simulink subsystem "subsistema_motores_bueno"  (R2023b)
settings: Solver=VariableStepAuto  StartTime=0.0  StopTime=10.0  RelTol=1e-3
libraries: arduinolib x6
settings Model: Creator=Usuario_UMA  LastModifiedBy=Usuario_UMA

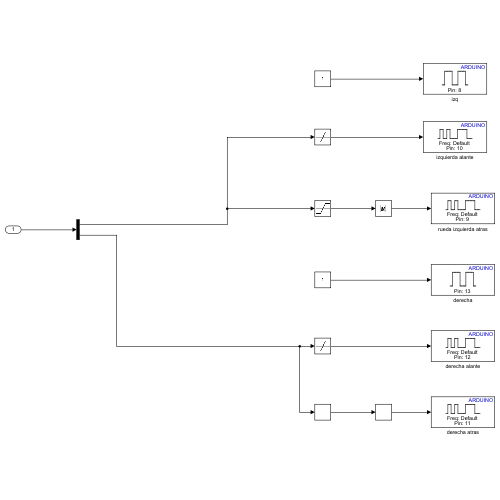
[thumbnail: Simulink's stored preview of the top-level diagram]
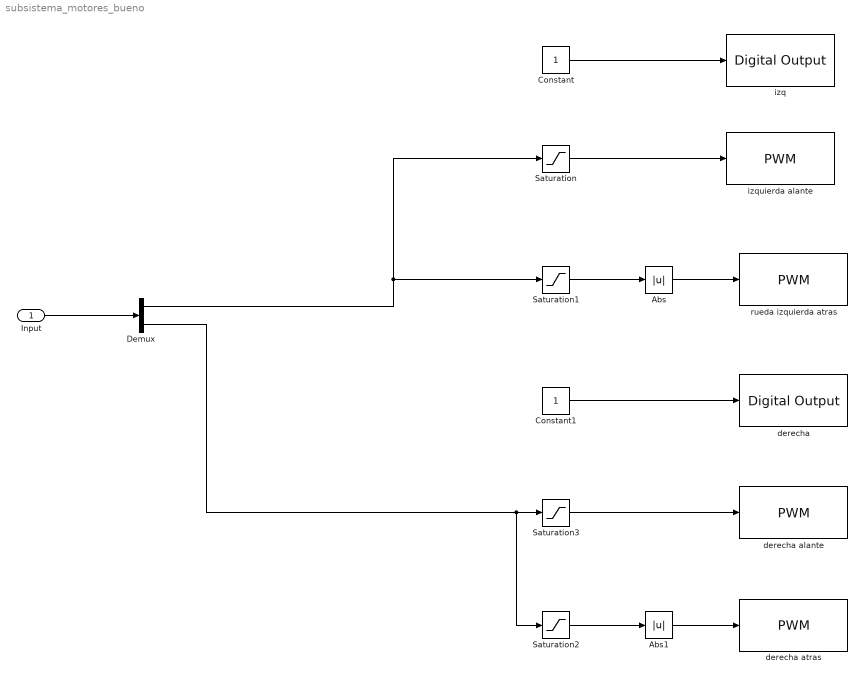
== system subsistema_motores_bueno ==
  Input : Inport
  Abs : Abs  SaturateOnIntegerOverflow=off
  Abs1 : Abs  SaturateOnIntegerOverflow=off
  Constant : Constant
  Constant1 : Constant
  Demux : Demux  Outputs=2
  Saturation : Saturate  UpperLimit=255  LowerLimit=0
  Saturation1 : Saturate  UpperLimit=0  LowerLimit=-255
  Saturation2 : Saturate  UpperLimit=0  LowerLimit=-255
  Saturation3 : Saturate  UpperLimit=255  LowerLimit=0
  derecha : arduinolib/Digital Output  pinNumber=13  Direction=output  blockPlatform=arduino
  derecha alante : arduinolib/PWM  pinNumber=12  frequencyType=Default  desiredFrequency=490.2  achievableFrequency=490.2
  derecha atras : arduinolib/PWM  pinNumber=11  frequencyType=Default  desiredFrequency=490.2  achievableFrequency=490.2
  izq : arduinolib/Digital Output  pinNumber=8  Direction=output  blockPlatform=arduino
  izquierda alante : arduinolib/PWM  pinNumber=10  frequencyType=Default  desiredFrequency=490.2  achievableFrequency=490.2
  rueda izquierda atras : arduinolib/PWM  pinNumber=9  frequencyType=Default  desiredFrequency=490.2  achievableFrequency=490.2
  wires:
  Saturation/1 -> izquierda alante/1
  Abs/1 -> rueda izquierda atras/1
  Demux/2 -> Saturation2/1, Saturation3/1
  Input/1 -> Demux/1
  Demux/1 -> Saturation/1, Saturation1/1
  Saturation1/1 -> Abs/1
  Saturation3/1 -> derecha alante/1
  Constant/1 -> izq/1
  Abs1/1 -> derecha atras/1
  Constant1/1 -> derecha/1
  Saturation2/1 -> Abs1/1
